simulink model "ADRC_Quanser"  (R2024a)
settings: Solver=ode1be  StartTime=0.0  StopTime=10  FixedStep=0.01  RelTol=1e-3
values from neighbouring files (symbols this model uses):
  l = 0.127    [Forward_Dynamics.m]    (also in Forward_Dynamics_ODE.m; Inverse_Dynamics.m)
  omega_c = 10^(omega_c_range(j))    [Strojenie.m]    (also in Wykresy3D.m = 0.5*(omega_c_ISE + omega_c_IAE))
  q0 = [0; -l/2; 3/2*pi; l/2; -l; 0; l; -l/2; pi/2; 3/2*l;0;0;-L; l; -l]    [Forward_Dynamics.m]    (also in Forward_Dynamics_ODE.m = [0; -l/2; 3/2*pi;      l/2; -l; 0;     l; -l/2; pi/2;      3; Inverse_Dynamics.m = [0; -l/2; 3/2*pi; l/2; -l; 0; l; -l/2; pi/2; 3/2*l;0;0;-L; l)
undefined symbols (not defined in the file or in its folder): Pk
libraries: slctrl_adaptive x2
settings Model: Creator=janek  LastModifiedBy=janek

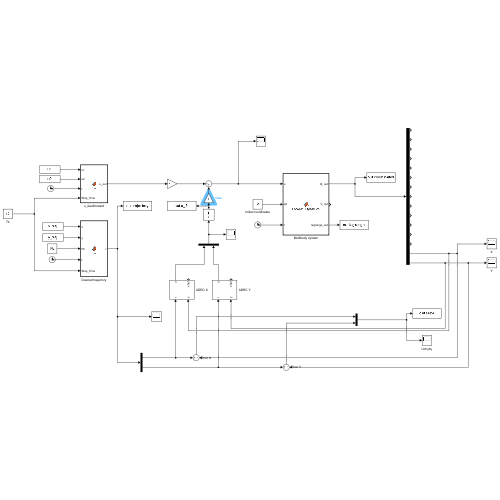
[thumbnail: Simulink's stored preview of the top-level diagram]
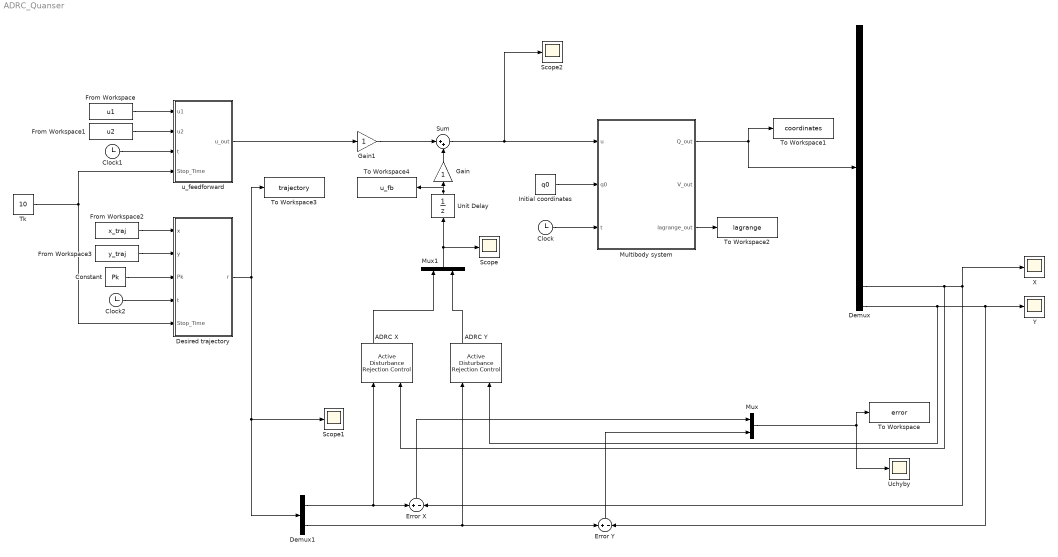
== system ADRC_Quanser ==
  ADRC X : slctrl_adaptive/Active Disturbance Rejection Control  time_domain=discrete-time  Ts=0.01  model_type=second-order  b0=b_hat  wc=omega_c  wo=omega_c*10  x0=[l;0;0]  ulim_checkbox=off  umax=inf  umin=-inf  xhat_checkbox=on
      settings: LibrarySourceBlock=slctrlblks/Adaptive Control/Active Disturbance Rejection Control
  ADRC Y : slctrl_adaptive/Active Disturbance Rejection Control  time_domain=discrete-time  Ts=0.01  model_type=second-order  b0=b_hat  wc=omega_c  wo=omega_c*10  x0=[-l;0;0]  ulim_checkbox=off  umax=inf  umin=-inf  xhat_checkbox=on
      settings: LibrarySourceBlock=slctrlblks/Adaptive Control/Active Disturbance Rejection Control
  Clock : Clock
  Clock1 : Clock
  Clock2 : Clock
  Constant : Constant  Value=Pk
  Demux : Demux  Outputs=15
  Demux1 : Demux  Outputs=2
  Desired trajectory : MATLAB Function  TreatAsAtomicUnit=on
  Error X : Sum  Inputs=+|-
  Error Y : Sum  Inputs=+|-
  From Workspace : FromWorkspace  VariableName=u1  OutDataTypeStr=double  SampleTime=0.01
  From Workspace1 : FromWorkspace  VariableName=u2
  From Workspace2 : FromWorkspace  VariableName=x_traj
  From Workspace3 : FromWorkspace  VariableName=y_traj
  Gain : Gain
  Gain1 : Gain
  Initial coordinates : Constant  Value=q0
  Multibody system : MATLAB Function  TreatAsAtomicUnit=on
  Mux : Mux  Inputs=2
  Mux1 : Mux  Inputs=2
  Scope : Scope
  Scope1 : Scope
  Scope2 : Scope
  Sum : Sum  Inputs=|++
  Tk : Constant  Value=10
  To Workspace : ToWorkspace  VariableName=error  SaveFormat=Timeseries  SampleTime=-1
  To Workspace1 : ToWorkspace  VariableName=coordinates  SaveFormat=Timeseries  SampleTime=-1
  To Workspace2 : ToWorkspace  VariableName=lagrange  SaveFormat=Timeseries  SampleTime=-1
  To Workspace3 : ToWorkspace  VariableName=trajectory  SaveFormat=Timeseries  SampleTime=-1
  To Workspace4 : ToWorkspace  VariableName=u_fb  SaveFormat=Timeseries  SampleTime=-1
  Uchyby : Scope
  Unit Delay : UnitDelay  SampleTime=-1  HasFrameUpgradeWarning=on
  X : Scope
  Y : Scope
  u_feedforward : MATLAB Function  TreatAsAtomicUnit=on
  wires:
  Initial coordinates/1 -> Multibody system/2(q0)
  Multibody system/1(Q_out) -> To Workspace1/1, Demux/1
  Demux/15 -> Y/1, Error Y/2, ADRC Y/2
  Demux/14 -> ADRC X/2, X/1, Error X/2
  Multibody system/3(lagrange_out) -> To Workspace2/1
  Sum/1 -> Scope2/1, Multibody system/1(u)
  Demux1/1 -> Error X/1, ADRC X/1
  Demux1/2 -> Error Y/1, ADRC Y/1
  Mux/1 -> Uchyby/1, To Workspace/1
  Clock1/1 -> u_feedforward/3(t)
  From Workspace/1 -> u_feedforward/1(u1)
  From Workspace1/1 -> u_feedforward/2(u2)
  From Workspace2/1 -> Desired trajectory/1(x)
  From Workspace3/1 -> Desired trajectory/2(y)
  Clock2/1 -> Desired trajectory/4(t)
  Desired trajectory/1(r) -> Demux1/1, Scope1/1, To Workspace3/1
  Constant/1 -> Desired trajectory/3(Pk)
  Error Y/1 -> Mux/2
  Error X/1 -> Mux/1
  u_feedforward/1(u_out) -> Gain1/1
  Tk/1 -> u_feedforward/4(Stop_Time), Desired trajectory/5(Stop_Time)
  Mux1/1 -> Unit Delay/1, Scope/1
  ADRC X/1 -> Mux1/1
  ADRC Y/1 -> Mux1/2
  Unit Delay/1 -> To Workspace4/1, Gain/1
  Clock/1 -> Multibody system/3(t)
  Gain/1 -> Sum/2
  Gain1/1 -> Sum/1

== matlab function ADRC_Quanser/Desired trajectory ==
  data: x input; r output; y input; Pk input; t input; Stop_Time input
function r = fcn(x, y, Pk, t, Stop_Time)
if t == Stop_Time   
    r = [Pk(1);Pk(2)];
else
    r = [x(round(t*100 + 1)); y(round(100*t + 1))];
end

== matlab function ADRC_Quanser/Multibody system ==
  settings: updateMethod=DISCRETE
  data: u input; Q_out output; q0 input; V_out output; lagrange_out output; t input
function [Q_out, V_out, lagrange_out] = Forward_Dynamics(u, q0, t)
l = 0.127;
L = l*2;
m1 = 0.065;
m2 = 0.5*m1;
J = 9.5e-5;
g = 9.81;
M = 1.2*diag([m1,m1,J, m1,m1,J, m1,m1,J, m1,m1,J, m2,m2,m2]);

q0 = q0(1:13);
persistent initial_guess;

if isempty(initial_guess)
        % Initialize at first call
        initial_guess = [q0;l;-l; zeros(26,1)]; 
end


options = optimoptions('fsolve', 'Algorithm', 'levenberg-marquardt','FunctionTolerance', 1e-10);

func = @(unknowns)FD(unknowns, initial_guess(1:15),initial_guess(16:30),u,M,l,L,t);
solution = fsolve(func, initial_guess, options);
initial_guess = solution; % Update the guess for the next call

Q_out = solution(1:15);
V_out = solution(16:30);
lagrange_out = solution(31:end);


function solution = FD(unknowns, q, v, u, M, l, L, t)
Q = unknowns(1:15);
V = unknowns(16:30);
Lag = unknowns(31:end);

m2 = M(13,13);
g = 9.81;
dt = 0.01;



Wiatr = 0;
%WIATR
if t >= 3 && t <=3.5
    Wiatr = m2*g/100;
end

F = [0;0;u(1); 0;0;0; 0;0;0; 0;0;u(2); -m2*g;0;0];
C = Phiq(Q(1:13),Q(14:15),l);
wiezy = Phi(Q(1:13),Q(14:15),l,L);

alpha = 100;
beta = 100;

A = [M C'; C zeros(11,11)];
b = [F;Gamma(Q,V,l) - 2*alpha*C*V - beta^2*wiezy];
x = A\b;

a = x(1:15);
lagrange = x(16:end);

solution = [
V - (Q - q)/dt;
a - (V - v)/dt;
Lag - lagrange;
];

end

function jakobi = Phiq(q,p,l)
q3 = q(3);
q6 = q(6);
q9 = q(9);
q12 = q(12);
q13 = q(13);
p1 = p(1);
p2 = p(2);

jakobi=[
[-1,  0,                                                                                                                                                             -(l*sin(q3))/2,  0,  0,                                                                                                                                                                          0,  0,  0,              0,  0,  0,               0,                                                                                   0,                                                                                                                       0,                                                                                                                       0]
[ 0, -1,                                                                                                                                                              (l*cos(q3))/2,  0,  0,                                                                                                                                                                          0,  0,  0,              0,  0,  0,               0,                                                                                   0,                                                                                                                       0,                                                                                                                       0]
[ 0,  0,                                                                                                                                                                 -l*sin(q3), -1,  0,                                                                                                                                                             -(l*sin(q6))/2,  0,  0,              0,  0,  0,               0,                                                                                   0,                                                                                                                       0,                                                                                                                       0]
[ 0,  0,                                                                                                                                                                  l*cos(q3),  0, -1,                                                                                                                                                              (l*cos(q6))/2,  0,  0,              0,  0,  0,               0,                                                                                   0,                                                                                                                       0,                                                                                                                       0]
[ 0,  0,                                                                                                                                                                 -l*sin(q3),  0,  0,                                                                                                                                                                 -l*sin(q6), -1,  0, -(l*sin(q9))/2,  0,  0,               0,                                                                                   0,                                                                                                                       0,                                                                                                                       0]
[ 0,  0,                                                                                                                                                                  l*cos(q3),  0,  0,                                                                                                                                                                  l*cos(q6),  0, -1,  (l*cos(q9))/2,  0,  0,               0,                                                                                   0,                                                                                                                       0,                                                                                                                       0]
[ 0,  0,                                                                                                                                                                 -l*sin(q3),  0,  0,                                                                                                                                                                 -l*sin(q6),  0,  0,     -l*sin(q9), -1,  0, -(l*sin(q12))/2,                                                                                   0,                                                                                                                       0,                                                                                                                       0]
[ 0,  0,                                                                                                                                                                  l*cos(q3),  0,  0,                                                                                                                                                                  l*cos(q6),  0,  0,      l*cos(q9),  0, -1,  (l*cos(q12))/2,                                                                                   0,                                                                                                                       0,                                                                                                                       0]
[ 0,  0,                                                                                                                                                                 -l*sin(q3),  0,  0,                                                                                                                                                                 -l*sin(q6),  0,  0,     -l*sin(q9),  0,  0,     -l*sin(q12),                                                                                   0,                                                                                                                       0,                                                                                                                       0]
[ 0,  0,                                                                                                                                                                  l*cos(q3),  0,  0,                                                                                                                                                                  l*cos(q6),  0,  0,      l*cos(q9),  0,  0,      l*cos(q12),                                                                                   0,                                                                                                                       0,                                                                                                                       0]
[ 0,  0, -(2*l*sin(q3)*(l*cos(q3) - p1 + l*cos(q6)) - 2*l*cos(q3)*(l*sin(q3) - p2 + l*sin(q6)))/(2*((l*cos(q3) - p1 + l*cos(q6))^2 + q13^2 + (l*sin(q3) - p2 + l*sin(q6))^2)^(1/2)),  0,  0, -(2*l*sin(q6)*(l*cos(q3) - p1 + l*cos(q6)) - 2*l*cos(q6)*(l*sin(q3) - p2 + l*sin(q6)))/(2*((l*cos(q3) - p1 + l*cos(q6))^2 + q13^2 + (l*sin(q3) - p2 + l*sin(q6))^2)^(1/2)),  0,  0,              0,  0,  0,               0, q13/((l*cos(q3) - p1 + l*cos(q6))^2 + q13^2 + (l*sin(q3) - p2 + l*sin(q6))^2)^(1/2), -(2*l*cos(q3) - 2*p1 + 2*l*cos(q6))/(2*((l*cos(q3) - p1 + l*cos(q6))^2 + q13^2 + (l*sin(q3) - p2 + l*sin(q6))^2)^(1/2)), -(2*l*sin(q3) - 2*p2 + 2*l*sin(q6))/(2*((l*cos(q3) - p1 + l*cos(q6))^2 + q13^2 + (l*sin(q3) - p2 + l*sin(q6))^2)^(1/2))]
 
];
end

function wiezy = Phi(q,p,l,L)
q1 = q(1);
q2 = q(2);
q3 = q(3);
q4 = q(4);
q5 = q(5);
q6 = q(6);
q7 = q(7);
q8 = q(8);
q9 = q(9);
q10 = q(10);
q11 = q(11);
q12 = q(12);
q13 = q(13);
p1 = p(1);
p2 = p(2);

wiezy =[

 
                                                                 (l*cos(q3))/2 - q1;
                                                                 (l*sin(q3))/2 - q2;
                                                     l*cos(q3) - q4 + (l*cos(q6))/2;
                                                     l*sin(q3) - q5 + (l*sin(q6))/2;
                                         l*cos(q3) - q7 + l*cos(q6) + (l*cos(q9))/2;
                                         l*sin(q3) - q8 + l*sin(q6) + (l*sin(q9))/2;
                           l*cos(q3) - q10 + l*cos(q6) + l*cos(q9) + (l*cos(q12))/2;
                           l*sin(q3) - q11 + l*sin(q6) + l*sin(q9) + (l*sin(q12))/2;
                               l*cos(q3) - 2*l + l*cos(q6) + l*cos(q9) + l*cos(q12);
                                     l*sin(q3) + l*sin(q6) + l*sin(q9) + l*sin(q12);
((l*cos(q3) - p1 + l*cos(q6))^2 + q13^2 + (l*sin(q3) - p2 + l*sin(q6))^2)^(1/2) - L;
];
 
                                                                
end

end

== matlab function ADRC_Quanser/u_feedforward ==
  data: u1 input; u2 input; u_out output; t input; Stop_Time input
function u_out = fcn(u1, u2, t, Stop_Time)
if t == Stop_Time
    u_out = [0; 0];
else
u_out = [u1(round(t*100) + 1); u2(round(t*100) + 1)];
end
